simulink model "ARDroneHoverSim_Pitch_2019"  (R2019a)
settings: Solver=ode1  StartTime=0.0  StopTime=300  FixedStep=simDT  RelTol=1e-3  EnableMultiTasking=on
undefined symbols (not defined in the file or in its folder): FMS
libraries: ARBlocks x3, aerolibanimutils x1, dspswit3 x1
settings Model: Creator=Paul Freeman  LastModifiedBy=Gaming
settings SolverCC: AutoInsertRateTranBlk=on
settings DataIOCC: SaveFormat=Array  SignalLoggingSaveFormat=ModelDataLogs  SaveOutput=off  SignalLogging=off  ReturnWorkspaceOutputs=off
settings OptimizationCC: ExpressionDepthLimit=2147483647  LifeSpan=inf
settings DebuggingCC: UnderspecifiedInitializationDetection=Classic  MergeDetectMultiDrivingBlocksExec=none  SolverPrmCheckMsg=warning  MultiTaskDSMMsg=warning  MultiTaskCondExecSysMsg=none  FcnCallInpInsideContextMsg=warning  StateNameClashWarn=warning  SFUnexpectedBacktrackingDiag=warning  SFNoUnconditionalDefaultTransitionDiag=warning  SFExecutionAtInitializationDiag=none  ArithmeticOperatorsInVariantConditions=warning
settings HardwareCC: ProdBitPerPointer=32  ProdBitPerSizeT=32  ProdBitPerPtrDiffT=32  ProdLargestAtomicInteger=Long  ProdLargestAtomicFloat=Double  ProdEndianess=BigEndian  ProdWordSize=32  ProdHWDeviceType=Freescale->32-bit PowerPC
settings ModelReferenceCC: PropagateSignalLabelsOutOfModel=off
settings SFSimCC: SimUseLocalCustomCode=off  SimParseCustomCode=off
settings RTWCC: RTWUseLocalCustomCode=off
settings CodeAppCC: StateflowObjectComments=on
settings GRTTargetCC: TargetLangStandard=C89/C90 (ANSI)  GeneratePreprocessorConditionals=Disable all  CombineOutputUpdateFcns=off  GRTInterface=on
settings ConfigComp: CovMetricSettings=dw  CovHtmlReporting=on  CovSaveCumulativeToWorkspaceVar=on  CovSaveSingleToWorkspaceVar=on  CovExternalEMLEnable=off

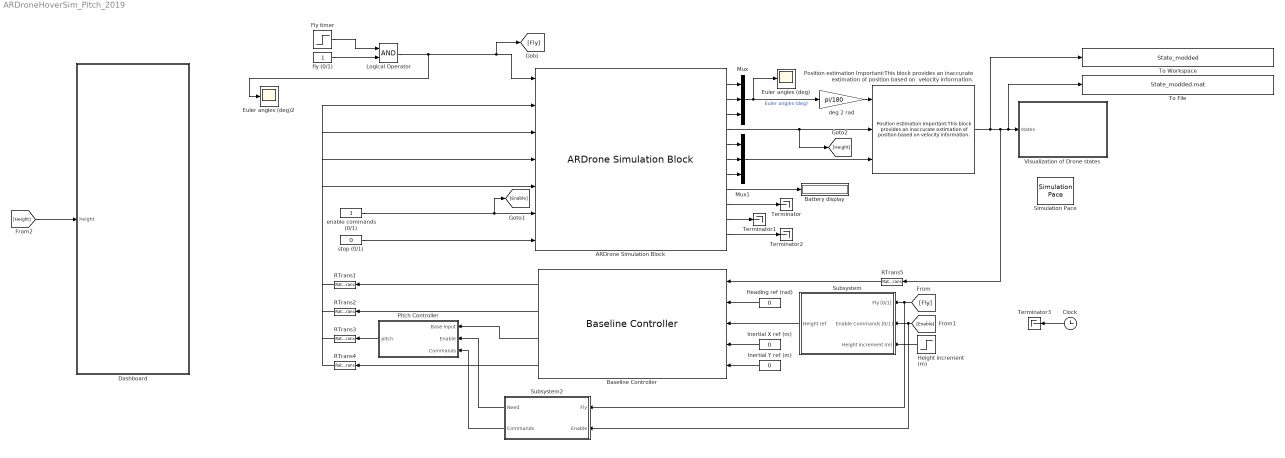
== system ARDroneHoverSim_Pitch_2019 ==
  ARDrone Simulation Block : ARBlocks/ARDrone Simulation Block  SystemSampleTime=-1
  Baseline Controller : ARBlocks/Baseline Controller  SystemSampleTime=-1
  Battery display : Display
  Clock : Clock
  Dashboard : Subsystem
  Euler angles (deg) : Scope
  Euler angles (deg)2 : Scope
  Fly timer : Step  Time=10
  Heading ref (rad) : Constant  Value=0  SampleTime=FMS.Ts
  Height increment (m) : Step  Time=15  After=0
  Inertial X ref (m) : Constant  Value=0  SampleTime=FMS.Ts
  Inertial Y ref (m) : Constant  Value=0  SampleTime=FMS.Ts
  Logical Operator : Logic  AllPortsSameDT=off  OutDataTypeStr=boolean
  Mux : Mux  Inputs=3
  Mux1 : Mux  Inputs=3
  Pitch Controller : Subsystem
  "Position estimation Important:This block provides an inaccurate extimation of position based on  velocity information. " : ARBlocks/Position estimation Important:This block provides an  inaccurate extimation of position  based on  velocity information.   SystemSampleTime=-1
  RTrans{1..4} (4 alike) : RateTransition  OutPortSampleTime=simDT
  RTrans5 : RateTransition  OutPortSampleTime=FMS.Ts
  Simulation Pace : aerolibanimutils/Simulation Pace  SimulationPace=1  SleepMode=MATLAB Thread  OutputPaceError=off  SampleTime=-1
  Subsystem : Subsystem
  Subsystem2 : Subsystem
  Terminator{,1..3} (4 alike) : Terminator
  To File : ToFile  Filename=State_modded.mat
  To Workspace : ToWorkspace  VariableName=State_modded  SaveFormat=Structure With Time  SampleTime=-1
      settings: Save2DSignal=2-D array (concatenate along first dimension)
  Visualization of Drone states : Subsystem
  deg 2 rad : Gain  Gain=pi/180
  enable commands (0/1) : Constant
  fly (0/1) : Constant
  stop (0/1) : Constant  Value=0
  wires:
  fly (0/1)/1 -> Logical Operator/2
  enable commands (0/1)/1 -> [Enable], ARDrone Simulation Block/6
  stop (0/1)/1 -> ARDrone Simulation Block/7
  ARDrone Simulation Block/1 -> Mux/1
  ARDrone Simulation Block/2 -> Mux/2
  ARDrone Simulation Block/5 -> Mux1/1
  ARDrone Simulation Block/6 -> Mux1/2
  ARDrone Simulation Block/7 -> Mux1/3
  Mux/1 -> deg 2 rad/1, Euler angles (deg)/1  "Euler angles (deg)"
  ARDrone Simulation Block/8 -> Battery display/1
  Baseline Controller/1 -> RTrans1/1
  "Position estimation Important:This block provides an inaccurate extimation of position based on  velocity information. "/1 -> To Workspace/1, RTrans5/1, To File/1, Visualization of Drone states/1(states)
  deg 2 rad/1 -> "Position estimation Important:This block provides an inaccurate extimation of position based on  velocity information. "/1
  ARDrone Simulation Block/4 -> [Height], "Position estimation Important:This block provides an inaccurate extimation of position based on  velocity information. "/2
  Mux1/1 -> "Position estimation Important:This block provides an inaccurate extimation of position based on  velocity information. "/3
  Baseline Controller/2 -> RTrans2/1
  Baseline Controller/4 -> RTrans4/1
  ARDrone Simulation Block/3 -> Mux/3
  ARDrone Simulation Block/9 -> Terminator/1
  RTrans1/1 -> ARDrone Simulation Block/5
  RTrans2/1 -> ARDrone Simulation Block/4
  RTrans3/1 -> ARDrone Simulation Block/3
  RTrans4/1 -> ARDrone Simulation Block/2
  ARDrone Simulation Block/10 -> Terminator1/1
  ARDrone Simulation Block/11 -> Terminator2/1
  Heading ref (rad)/1 -> Baseline Controller/2
  Inertial X ref (m)/1 -> Baseline Controller/4
  Inertial Y ref (m)/1 -> Baseline Controller/5
  RTrans5/1 -> Baseline Controller/1
  [Fly] -> Subsystem2/1(Fly), Subsystem/1(Fly [0/1])
  [Enable] -> Subsystem/2(Enable Commands [0/1]), Subsystem2/2(Enable)
  Height increment (m)/1 -> Subsystem/3(Height increment (m))
  Subsystem/1(Height ref) -> Baseline Controller/3
  Clock/1 -> Terminator3/1
  Fly timer/1 -> Logical Operator/1
  Logical Operator/1 -> Euler angles (deg)2/1, ARDrone Simulation Block/1, [Fly]
  [Height] -> Dashboard/1(height)
  Baseline Controller/3 -> Pitch Controller/1(Base Input)
  Pitch Controller/1(pitch) -> RTrans3/1
  Subsystem2/1(Need) -> Pitch Controller/2(Enable)
  Subsystem2/2(Commands) -> Pitch Controller/3(Commands)

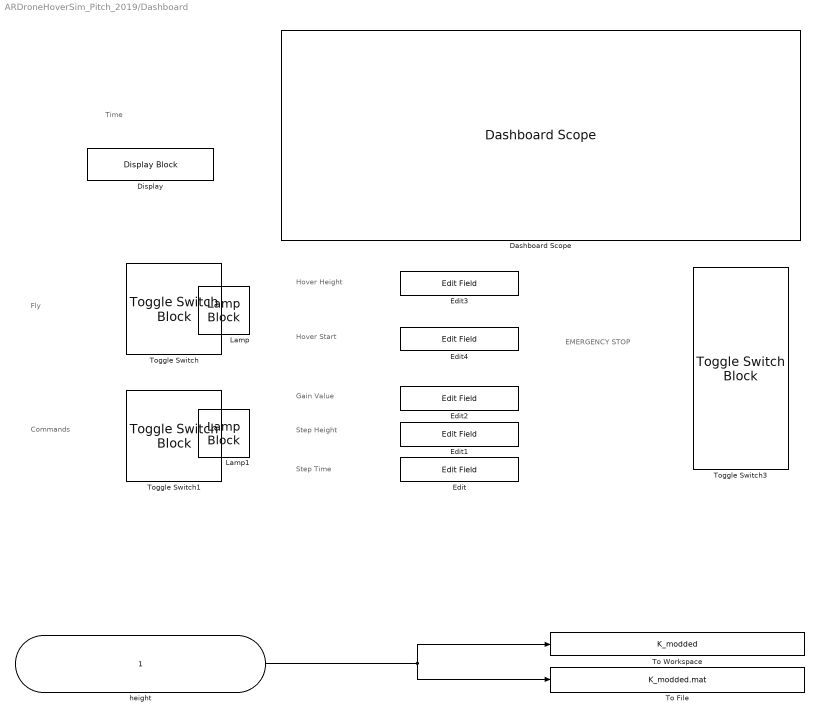
== system ARDroneHoverSim_Pitch_2019/Dashboard ==
  note: Fly
  note: Commands
  note: EMERGENCY
      | STOP
  note: Step Height
  note: Step Time
  note: Gain Value
  note: Time
  note: Hover Start
  note: Hover Height
  height : Inport
  Dashboard Scope : DashboardScope  Ymin=-2  Ymax=2
  Display : DisplayBlock  LabelPosition=Hide  Format=short
  Edit{,1..4} (5 alike) : EditField  LabelPosition=Hide  ShowInitialText=on  Alignment=Center
  Lamp : LampBlock  LabelPosition=Hide
  Lamp1 : LampBlock  LabelPosition=Hide
  To File : ToFile  Filename=K_modded.mat
  To Workspace : ToWorkspace  VariableName=K_modded  SaveFormat=Structure With Time  SampleTime=-1
      settings: Save2DSignal=2-D array (concatenate along first dimension)
  Toggle Switch : ToggleSwitchBlock  LabelPosition=Hide
      settings: Values={{'Land', 'Take Off'}, [0 1]}
  Toggle Switch1 : ToggleSwitchBlock  LabelPosition=Hide
      settings: Values={{'Disable', 'Enable'}, [0 1]}
  Toggle Switch3 : ToggleSwitchBlock  LabelPosition=Hide
      settings: Values={{'-', '-'}, [0 1]}
  wires:
  height/1 -> To File/1, To Workspace/1

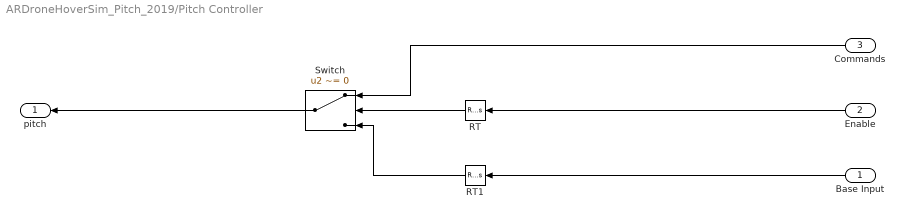
== system ARDroneHoverSim_Pitch_2019/Pitch Controller ==
  Base Input : Inport
  Enable : Inport  Port=2
  Commands : Inport  Port=3
  RT : RateTransition  OutPortSampleTime=0.005
  RT1 : RateTransition  OutPortSampleTime=0.005
  Switch : Switch  Criteria=u2 ~= 0
  pitch : Outport
  wires:
  Base Input/1 -> RT1/1
  RT/1 -> Switch/2
  Commands/1 -> Switch/1
  RT1/1 -> Switch/3
  Switch/1 -> pitch/1
  Enable/1 -> RT/1

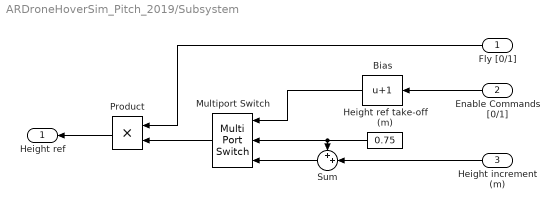
== system ARDroneHoverSim_Pitch_2019/Subsystem ==
  Fly [0/1] : Inport
  Enable Commands [0/1] : Inport  Port=2
  Height increment (m) : Inport  Port=3
  Bias : Bias  Bias=1
  Height ref take-off (m) : Constant  Value=0.75  SampleTime=FMS.Ts
  Multiport Switch : MultiPortSwitch  Inputs=2
  Product : Product
  Sum : Sum  Inputs=++|
  Height ref : Outport
  wires:
  Multiport Switch/1 -> Product/2
  Enable Commands [0/1]/1 -> Bias/1
  Fly [0/1]/1 -> Product/1
  Height ref take-off (m)/1 -> Sum/1, Multiport Switch/2
  Product/1 -> Height ref/1
  Height increment (m)/1 -> Sum/2
  Bias/1 -> Multiport Switch/1
  Sum/1 -> Multiport Switch/3

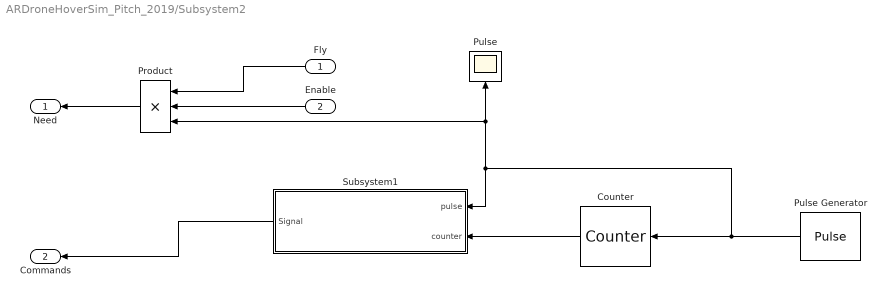
== system ARDroneHoverSim_Pitch_2019/Subsystem2 ==
  Fly : Inport
  Enable : Inport  Port=2
  Counter : dspswit3/Counter  Direction=Up  CountEvent=Rising edge  CounterSize=User defined  MaxCount=255  InitialCount=0  Output=Count  HitValue=32  ResetInput=off  SamplesPerFrame=1  Ts=1  CntDtype=double  HitDtype=Logical
  Product : Product  Inputs=3
  Pulse : Scope
  Pulse Generator : DiscretePulseGenerator  Period=1500  PulseWidth=1000  PhaseDelay=1000  SampleTime=0.03
  Subsystem1 : Subsystem
  Need : Outport
  Commands : Outport  Port=2
  wires:
  Counter/1 -> Subsystem1/2(counter)
  Pulse Generator/1 -> Counter/1, Product/3, Pulse/1, Subsystem1/1(pulse)
  Subsystem1/1(Signal) -> Commands/1
  Fly/1 -> Product/1
  Enable/1 -> Product/2
  Product/1 -> Need/1

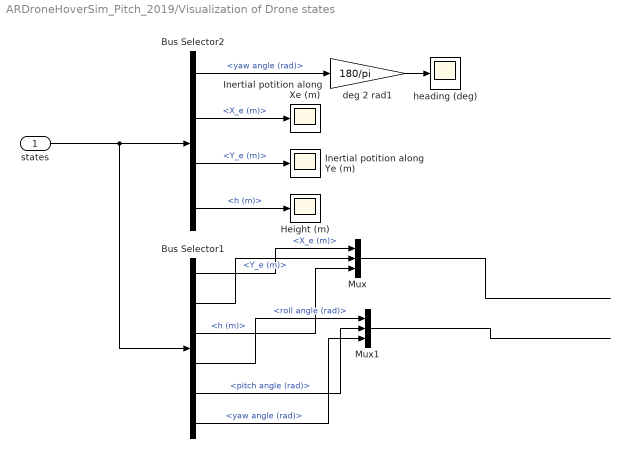
== system ARDroneHoverSim_Pitch_2019/Visualization of Drone states ==
  states : Inport
  Bus Selector1 : BusSelector  OutputSignals=X_e (m),Y_e (m),h (m),roll angle (rad),pitch angle (rad),yaw angle (rad)
  Bus Selector2 : BusSelector  OutputSignals=yaw angle (rad),X_e (m),Y_e (m),h (m)
  Height (m) : Scope
  Inertial potition along Xe (m) : Scope
  Inertial potition along Ye (m) : Scope
  Mux : Mux  Inputs=3
  Mux1 : Mux  Inputs=3
  deg 2 rad1 : Gain  Gain=180/pi
  heading (deg) : Scope
  wires:
  states/1 -> Bus Selector1/1, Bus Selector2/1
  Bus Selector2/1 -> deg 2 rad1/1  "<yaw angle (rad)>"
  Bus Selector2/2 -> Inertial potition along Xe (m)/1  "<X_e (m)>"
  Bus Selector2/3 -> Inertial potition along Ye (m)/1  "<Y_e (m)>"
  Bus Selector2/4 -> Height (m)/1  "<h (m)>"
  deg 2 rad1/1 -> heading (deg)/1
  Bus Selector1/1 -> Mux/1  "<X_e (m)>"
  Bus Selector1/2 -> Mux/2  "<Y_e (m)>"
  Bus Selector1/3 -> Mux/3  "<h (m)>"
  Mux/1 -> ?
  Bus Selector1/4 -> Mux1/1  "<roll angle (rad)>"
  Bus Selector1/5 -> Mux1/2  "<pitch angle (rad)>"
  Bus Selector1/6 -> Mux1/3  "<yaw angle (rad)>"
  Mux1/1 -> ?

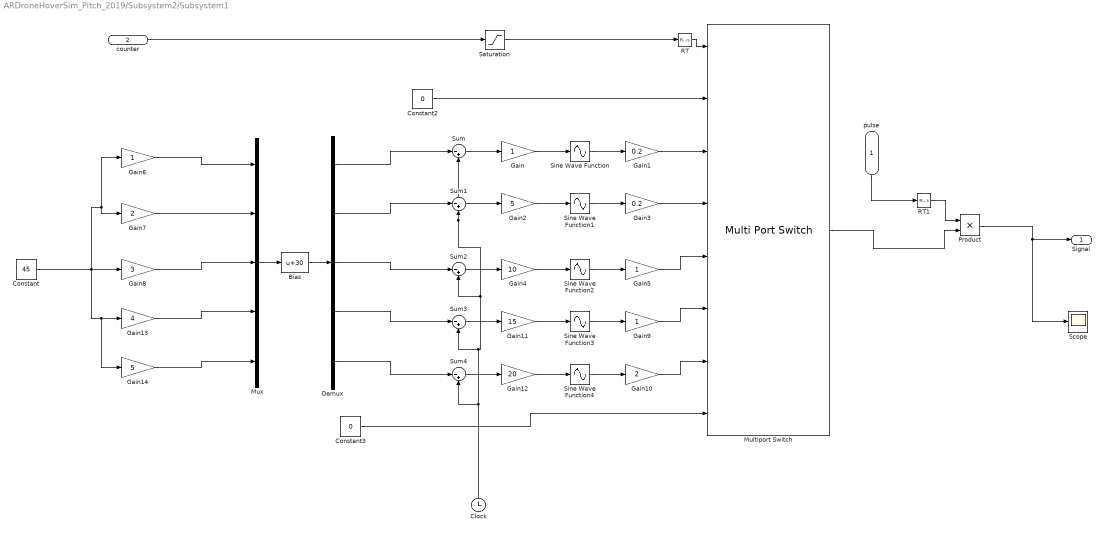
== system ARDroneHoverSim_Pitch_2019/Subsystem2/Subsystem1 ==
  pulse : Inport
  counter : Inport  Port=2
  Bias : Bias  Bias=30
  Clock : Clock
  Constant : Constant  Value=45
  Constant2 : Constant  Value=0
  Constant3 : Constant  Value=0
  Demux : Demux  Outputs=5
  Gain{,5..6,9} (4 alike) : Gain
  Gain1 : Gain  Gain=0.2
  Gain10 : Gain  Gain=2
  Gain11 : Gain  Gain=15
  Gain12 : Gain  Gain=20
  Gain13 : Gain  Gain=4
  Gain14 : Gain  Gain=5
  Gain2 : Gain  Gain=5
  Gain3 : Gain  Gain=0.2
  Gain4 : Gain  Gain=10
  Gain7 : Gain  Gain=2
  Gain8 : Gain  Gain=3
  Multiport Switch : MultiPortSwitch  DataPortOrder=Zero-based contiguous  Inputs=7  zeroidx=on
  Mux : Mux  Inputs=5
  Product : Product
  RT : RateTransition  OutPortSampleTime=0.005
  RT1 : RateTransition  OutPortSampleTime=0.005
  Saturation : Saturate  UpperLimit=6  LowerLimit=0
  Scope : Scope
  Sine Wave Function{,1..4} (5 alike) : Sin  TimeSource=Use external signal  SampleTime=0
  Sum{,1..4} (5 alike) : Sum  Inputs=|-+
  Signal : Outport
  wires:
  Gain4/1 -> Sine Wave Function2/1
  Sum1/1 -> Gain2/1
  Gain2/1 -> Sine Wave Function1/1
  Sine Wave Function/1 -> Gain1/1
  Gain/1 -> Sine Wave Function/1
  Sine Wave Function1/1 -> Gain3/1
  Sum2/1 -> Gain4/1
  Gain5/1 -> Multiport Switch/5
  Gain1/1 -> Multiport Switch/3
  Constant/1 -> Gain13/1, Gain14/1, Gain6/1, Gain7/1, Gain8/1
  Sine Wave Function2/1 -> Gain5/1
  Mux/1 -> Bias/1
  Sum/1 -> Gain/1
  Gain3/1 -> Multiport Switch/4
  Bias/1 -> Demux/1
  counter/1 -> Saturation/1
  Constant2/1 -> Multiport Switch/2
  Constant3/1 -> Multiport Switch/8
  Gain10/1 -> Multiport Switch/7
  Gain9/1 -> Multiport Switch/6
  Sine Wave Function3/1 -> Gain9/1
  Sine Wave Function4/1 -> Gain10/1
  Clock/1 -> Sum2/2, Sum1/2, Sum/2, Sum3/2, Sum4/2
  Demux/1 -> Sum/1
  Demux/2 -> Sum1/1
  Demux/3 -> Sum2/1
  Sum3/1 -> Gain11/1
  Gain12/1 -> Sine Wave Function4/1
  Sum4/1 -> Gain12/1
  Gain11/1 -> Sine Wave Function3/1
  Demux/4 -> Sum3/1
  Demux/5 -> Sum4/1
  Gain6/1 -> Mux/1
  Gain7/1 -> Mux/2
  Gain8/1 -> Mux/3
  Gain13/1 -> Mux/4
  Gain14/1 -> Mux/5
  Product/1 -> Scope/1, Signal/1
  Multiport Switch/1 -> Product/2
  pulse/1 -> RT1/1
  RT/1 -> Multiport Switch/1
  RT1/1 -> Product/1
  Saturation/1 -> RT/1
